simulink model "Model_Direct_design_controller_SS_robust_tracking_system"  (R2024b)
settings: Solver=VariableStepDiscrete  StartTime=0.0  StopTime=15  RelTol=1e-3
values from neighbouring files (symbols this model uses):
  K_I = K_stateFB_extended(:,1)    [Controller_SS_direct_design_control_vars_robusttracking.m]
  K_stateFB = K_stateFB_extended(:,2:3)    [Controller_SS_direct_design_control_vars_robusttracking.m]
  Nu = solution(3,:)    [Controller_SS_direct_design_control_vars_robusttracking.m]
  Nx = solution(1:2,:)    [Controller_SS_direct_design_control_vars_robusttracking.m]
  Ts = Ts_values(i)    [A_final_results.m]
undefined symbols (not defined in the file or in its folder): DiscIntNeverNeededParam, sigmaD_tf_den, sigmaD_tf_num
settings Model: Creator=Riccardo Grosso  LastModifiedBy=Buton

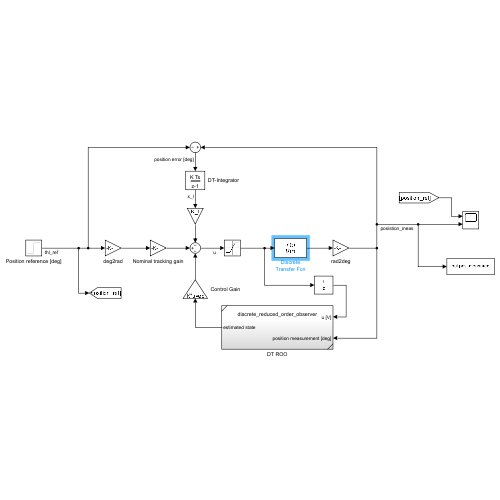
[thumbnail: Simulink's stored preview of the top-level diagram]
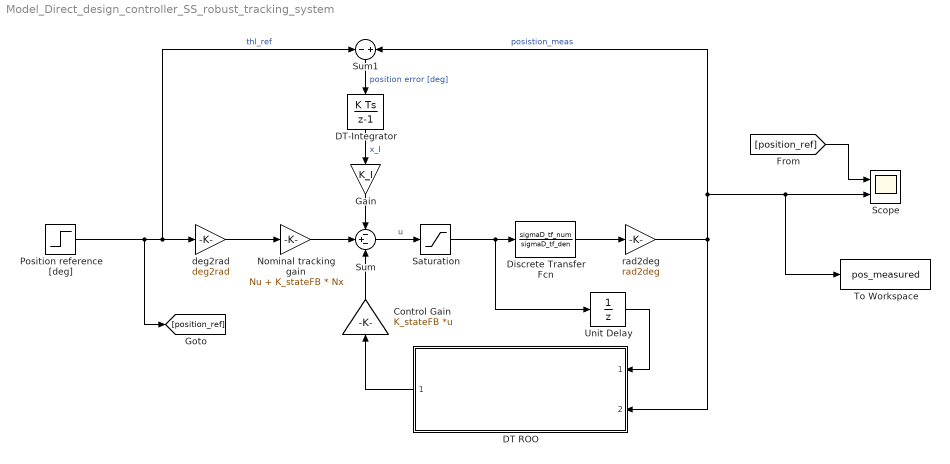
== system Model_Direct_design_controller_SS_robust_tracking_system ==
  Control Gain : Gain  Gain=K_stateFB  Multiplication=Matrix(K*u) (u vector)
  DT ROO : Subsystem  ReferencedSubsystem=discrete_reduced_order_observer
  DT-Integrator : DiscreteIntegrator  SampleTime=0.05  ICPrevOutput=DiscIntNeverNeededParam  ICPrevScaledInput=DiscIntNeverNeededParam
  Discrete Transfer Fcn : DiscreteTransferFcn  Numerator=sigmaD_tf_num  Denominator=sigmaD_tf_den
  Gain : Gain  Gain=K_I
  Nominal tracking gain : Gain  Gain=Nu + K_stateFB * Nx
  Position reference [deg] : Step  After=50  SampleTime=Ts
  Saturation : Saturate  UpperLimit=12  LowerLimit=-12
  Scope : Scope  NumInputPorts=2
  Sum : Sum  Inputs=-+-
  Sum1 : Sum  Inputs=-|+
  To Workspace : ToWorkspace  VariableName=pos_measured  SaveFormat=Timeseries  SampleTime=-1
  Unit Delay : UnitDelay  SampleTime=-1  HasFrameUpgradeWarning=on
  deg2rad : Gain  Gain=deg2rad
  rad2deg : Gain  Gain=rad2deg
  wires:
  rad2deg/1 -> To Workspace/1, Scope/2, Sum1/2, DT ROO/2  "posistion_meas"
  Discrete Transfer Fcn/1 -> rad2deg/1
  Sum/1 -> Saturation/1  "u"
  deg2rad/1 -> Nominal tracking gain/1
  Position reference [deg]/1 -> [position_ref], Sum1/1, deg2rad/1  "thl_ref"
  Saturation/1 -> Unit Delay/1, Discrete Transfer Fcn/1
  Nominal tracking gain/1 -> Sum/2
  Sum1/1 -> DT-Integrator/1  "position error [deg]"
  DT-Integrator/1 -> Gain/1  "x_I"
  Gain/1 -> Sum/1
  Control Gain/1 -> Sum/3
  DT ROO/1 -> Control Gain/1
  [position_ref] -> Scope/1
  Unit Delay/1 -> DT ROO/1
